simulink model "stellaris_test_blink"  (R2012b)
settings: Solver=FixedStepDiscrete  SolverMode=SingleTasking  StartTime=0.0  StopTime=10.0  FixedStep=0.2  RelTol=1e-3
libraries: stellaris_lib x5, simulink x2
settings Model: Creator=peselnikmg  LastModifiedBy=peselnikmg
settings DataIOCC: SignalLoggingSaveFormat=ModelDataLogs
settings OptimizationCC: OptimizeModelRefInitCode=on  LifeSpan=1
settings HardwareCC: ProdEndianess=LittleEndian  ProdHWDeviceType=Texas Instruments->TMS470
settings RTWCC: SystemTargetFile=stellaris.tlc  TemplateMakefile=stellaris_tmf  PostCodeGenCommand=stellaris_customcode(buildInfo)  Description=TI Stellaris LaunchPad  GenerateReport=on  ProcessScript=stellaris_make_rtw_hook  IncludeHyperlinkInReport=on  GenerateTraceInfo=on  GenerateTraceReport=on  GenerateTraceReportSl=on  GenerateTraceReportSf=on  GenerateTraceReportEml=on  GenerateCodeMetricsReport=on  GenerateCodeReplacementReport=on
settings CodeAppCC: IgnoreCustomStorageClasses=off
settings STFCustomTargetCC: CodeReplacementLibrary=ANSI_C  CombineOutputUpdateFcns=on  ERTCustomFileBanners=on  SupportContinuousTime=off  SupportNonInlinedSFcns=off  GRTInterface=off  SystemTargetFile=stellaris.tlc
settings ERTTargetCC: CodeReplacementLibrary=ANSI_C  MultiwordLength=2048  ParMdlRefBuildCompliant=off  CompOptLevelCompliant=off  ConcurrentExecutionCompliant=off  ERTFirstTimeCompliant=off  ModelStepFunctionPrototypeControlCompliant=off  CPPClassGenCompliant=off  InlinedParameterPlacement=NonHierarchical  ERTCustomFileTemplate=stellaris_srmain.tlc  ConvertIfToSwitch=off  SuppressUnreachableDefaultCases=off

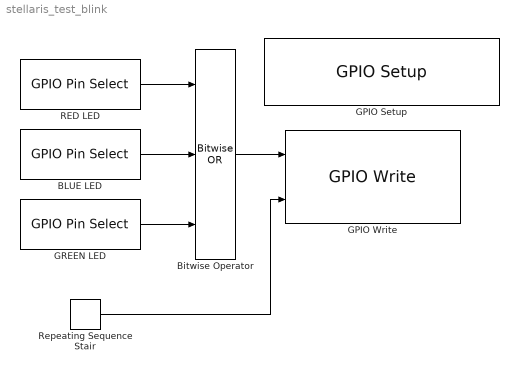
== system stellaris_test_blink ==
  BLUE LED : stellaris_lib/GPIO/GPIO Pin Select  GPIO_PIN_X=GPIO_PIN_2
  Bitwise Operator : simulink/Logic and Bit Operations/Bitwise Operator  logicop=OR  UseBitMask=off  NumInputPorts=3  BitMask=bin2dec('11011001')  BitMaskRealWorld=Stored Integer
  GPIO Setup : stellaris_lib/GPIO/GPIO Setup  GPIO_PORTX_BASE=GPIO_PORTF_BASE  PinsOutput_0=Input  PinsOutput_1=Output  PinsOutput_2=Output  PinsOutput_3=Output  PinsOutput_4=Input  PinsOutput_5=Input  PinsOutput_6=Input  PinsOutput_7=Input
  GPIO Write : stellaris_lib/GPIO/GPIO Write  GPIO_PORTX_BASE=GPIO_PORTF_BASE
  GREEN LED : stellaris_lib/GPIO/GPIO Pin Select  GPIO_PIN_X=GPIO_PIN_3
  RED LED : stellaris_lib/GPIO/GPIO Pin Select  GPIO_PIN_X=GPIO_PIN_1
  Repeating Sequence Stair : simulink/Sources/Repeating Sequence Stair  OutValues=[0 2 4 8].'  tsamp=1  OutMin=[]  OutMax=[]  OutDataTypeStr=uint8  OutputDataTypeScalingMode=uint8  OutDataType=fixdt(0,8)  ConRadixGroup=Best Precision: Vector-wise  OutScaling=2^-12
  wires:
  BLUE LED/1 -> Bitwise Operator/2
  RED LED/1 -> Bitwise Operator/1
  GREEN LED/1 -> Bitwise Operator/3
  Bitwise Operator/1 -> GPIO Write/1
  Repeating Sequence Stair/1 -> GPIO Write/2
